simulink model "motomatic_pend"  (R2020b)
settings: Solver=VariableStepAuto  StartTime=0.0  StopTime=10.0  RelTol=1e-7
undefined symbols (not defined in the file or in its folder): Ka, Kp, Kstar, Kt, N, physParam, th_init
settings Model: Creator=Bradley Kwan  LastModifiedBy=Bradley Kwan

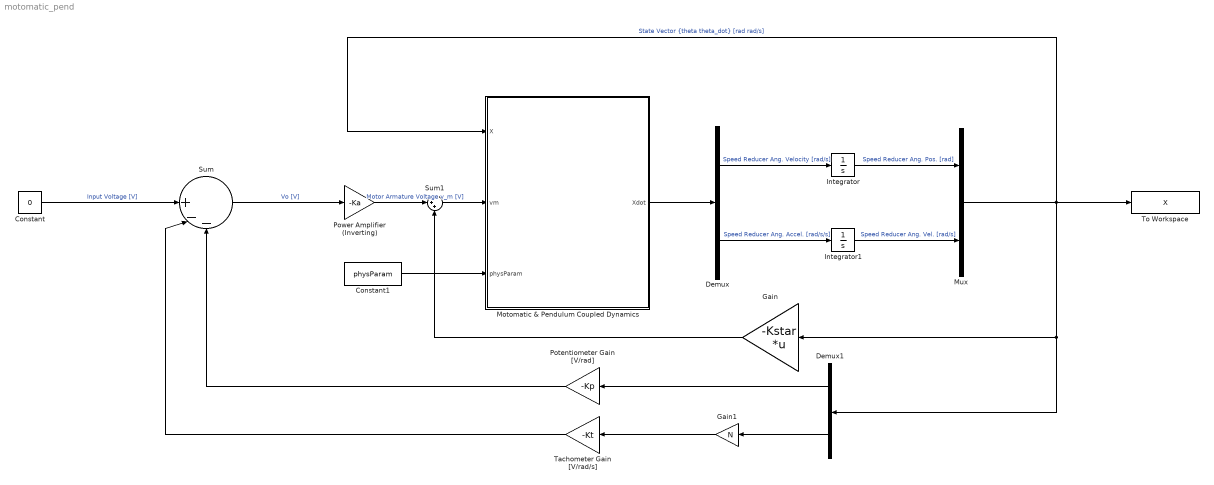
== system motomatic_pend ==
  Constant : Constant  Value=0
  Constant1 : Constant  Value=physParam
  Demux : Demux  Outputs=2
  Demux1 : Demux  Outputs=2
  Gain : Gain  Gain=-Kstar  Multiplication=Matrix(K*u)
  Gain1 : Gain  Gain=N
  Integrator : Integrator  InitialCondition=th_init
  Integrator1 : Integrator
  Motomatic & Pendulum Coupled Dynamics : MATLAB Function  TreatAsAtomicUnit=on
  Mux : Mux  Inputs=2
  Potentiometer Gain [V/rad] : Gain  Gain=-Kp
  Power Amplifier (Inverting) : Gain  Gain=-Ka
  Sum : Sum  Inputs=||+--
  Sum1 : Sum  Inputs=|++
  Tachometer Gain [V/rad/s] : Gain  Gain=-Kt
  To Workspace : ToWorkspace  VariableName=X  SampleTime=-1
  wires:
  Sum/1 -> Power Amplifier (Inverting)/1  "Vo [V]"
  Constant/1 -> Sum/1  "Input Voltage [V]"
  Constant1/1 -> Motomatic & Pendulum Coupled Dynamics/3(physParam)
  Motomatic & Pendulum Coupled Dynamics/1(Xdot) -> Demux/1
  Demux/1 -> Integrator/1  "Speed Reducer Ang. Velocity [rad/s]"
  Demux/2 -> Integrator1/1  "Speed Reducer Ang. Accel. [rad/s/s]"
  Integrator/1 -> Mux/1  "Speed Reducer Ang. Pos. [rad]"
  Integrator1/1 -> Mux/2  "Speed Reducer Ang. Vel. [rad/s]"
  Mux/1 -> To Workspace/1, Motomatic & Pendulum Coupled Dynamics/1(X), Demux1/1, Gain/1  "State Vector {theta theta_dot} [rad rad/s]"
  Demux1/2 -> Gain1/1
  Demux1/1 -> Potentiometer Gain [V/rad]/1
  Gain1/1 -> Tachometer Gain [V/rad/s]/1
  Potentiometer Gain [V/rad]/1 -> Sum/3
  Tachometer Gain [V/rad/s]/1 -> Sum/2
  Gain/1 -> Sum1/2
  Power Amplifier (Inverting)/1 -> Sum1/1  "Motor Armature Voltage v_m [V]"
  Sum1/1 -> Motomatic & Pendulum Coupled Dynamics/2(vm)

== matlab function motomatic_pend/Motomatic & Pendulum Coupled Dynamics ==
  data: X input; Xdot output; vm input; physParam input
function Xdot = motor_dynamics(X,vm, physParam)

% First define the physical parameters of the pendulum model
M = physParam(1);      % bob mass [kg]
L = physParam(2);      % pendulum length [m]
g = physParam(3);      % gravitational acceleration [m/s/s]
vmo = physParam(4);    % Voltage necessary to hold pendulum at 90 degrees [v]
N = physParam(5);      % speed reducer factor

% Based on the physical parameters of the model, find the polar moments of
% inertia of the motor and pendulum
J_p = M*L^2;                    % Polar moment inertia of pendulum [kg*m^2]
J_m = M*g*L/vmo*(.2740/19.763); % Polar moment inertia of motor [kg*m^2]

Xdot = [NaN NaN];

% First the function tests to see if the motor will overcome stiction
if abs(vm) < .8316 && X(2) == 0 
    Xdot = [0 0];
else
    % Assymetric friction function to determine tau_m F(x(1))
    tau_m = .274;    % using the linearized time constant for now...
    Xdot(1) = X(2);
    Xdot(2) = -N*J_m/tau_m/(N*J_m+J_p)*X(2) ...
              +M*g*L*sin(X(1))/(N*J_m+J_p) + ...
              M*g*L/(vmo*(N*J_m+J_p))*vm;
end
